simulink model "Sim_EX_03"  (R2017a)
settings: Solver=VariableStepAuto  StartTime=0.0  StopTime=1/60  MaxStep=1e-6  RelTol=1e-3
libraries: simulink x1
settings Model: Creator=KYC  LastModifiedBy=KYC

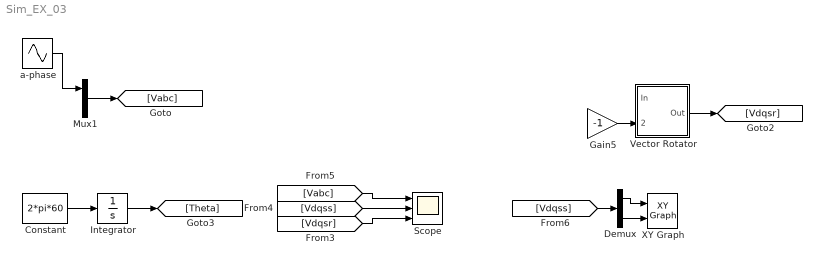
== system Sim_EX_03 ==
  Constant : Constant  Value=2*pi*60
  Demux : Demux  Outputs=2
  Gain5 : Gain  Gain=-1
  Integrator : Integrator
  Mux1 : Mux  Inputs=3
  Scope : Scope  NumInputPorts=3
  Vector Rotator : Subsystem
  XY Graph : simulink/Sinks/XY Graph  xmin=-200  xmax=200  ymin=-200  ymax=200  st=-1
  a-phase : Sin  Amplitude=220*sqrt(2)/sqrt(3)  Frequency=2*pi*60  Phase=pi  SampleTime=0
  wires:
  Gain5/1 -> Vector Rotator/2(Theta)
  a-phase/1 -> Mux1/1
  Mux1/1 -> [Vabc]
  Vector Rotator/1(Out) -> [Vdqsr]
  Constant/1 -> Integrator/1
  Integrator/1 -> [Theta]
  [Vdqss] -> Scope/2
  [Vabc] -> Scope/1
  [Vdqsr] -> Scope/3
  [Vdqss] -> Demux/1
  Demux/2 -> XY Graph/2
  Demux/1 -> XY Graph/1

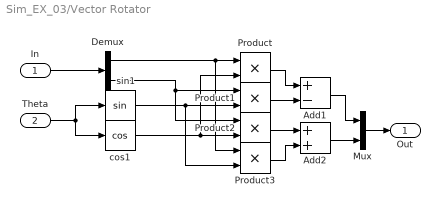
== system Sim_EX_03/Vector Rotator ==
  In : Inport
  Theta : Inport  Port=2
  Add1 : Sum  Inputs=+-
  Add2 : Sum
  Demux : Demux  Outputs=2
  Mux : Mux  Inputs=[1 1]
  Product{,1..3} (4 alike) : Product  RndMeth=Zero
  cos1 : Trigonometry  Operator=cos
  sin1 : Trigonometry
  Out : Outport
  wires:
  Theta/1 -> cos1/1, sin1/1
  Demux/1 -> Product3/1, Product/1
  Mux/1 -> Out/1
  In/1 -> Demux/1
  Demux/2 -> Product1/1, Product2/1
  cos1/1 -> Product/2, Product2/2
  sin1/1 -> Product1/2, Product3/2
  Product/1 -> Add1/1
  Product1/1 -> Add1/2
  Add1/1 -> Mux/1
  Product2/1 -> Add2/1
  Product3/1 -> Add2/2
  Add2/1 -> Mux/2
